simulink model "DinamicaCompleta"  (R2015a)
settings: Solver=ode45  StartTime=0.0  StopTime=10.0  RelTol=1e-3
values from neighbouring files (symbols this model uses):
  g = 1.6    [InitialParameters.m]
  M0 = 15000 - MFuel0    (= 7000)    [InitialParameters.m]
  MaxFl = 500    [InitialParameters.m]
  MaxFt = 44000    [InitialParameters.m]
  MFuel0 = 8000    [InitialParameters.m]
  Power = 3000    [InitialParameters.m]
  theta0 = 0    [InitialParameters.m]
  theta_dot0 = 0    [InitialParameters.m]
  x0 = 500    [InitialParameters.m]
  x_dot0 = 0    [InitialParameters.m]
  y0 = 160000    [InitialParameters.m]
  y_dot0 = -700    [InitialParameters.m]
settings Model: Creator=MateusVendramini  LastModifiedBy=MateusVendramini

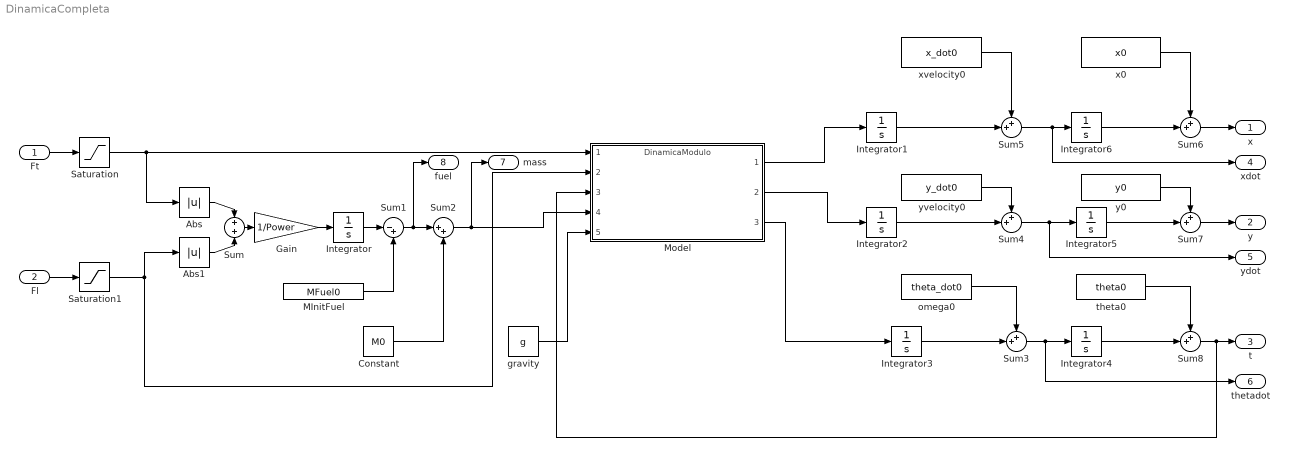
== system DinamicaCompleta ==
  Ft : Inport
  Fl : Inport  Port=2
  Abs : Abs
  Abs1 : Abs
  Constant : Constant  Value=M0
  Gain : Gain  Gain=1/Power
  Integrator{,1..6} (7 alike) : Integrator
  "MInitFuel " : Constant  Value=MFuel0
  Model : ModelReference  ModelNameDialog=DinamicaModulo.slx  SimulationMode=Normal  ModelReferenceVersion=1.3  CopyOfModelName=DinamicaModulo.slx  DefaultDataLogging=on
  Saturation : Saturate  UpperLimit=MaxFt  LowerLimit=-MaxFt
  Saturation1 : Saturate  UpperLimit=MaxFl  LowerLimit=-MaxFl
  Sum : Sum
  Sum1 : Sum  Inputs=|-+
  Sum2 : Sum  Inputs=|++
  Sum{3..8} (6 alike) : Sum  Inputs=++|
  gravity : Constant  Value=g
  omega0 : Constant  Value=theta_dot0
  theta0 : Constant  Value=theta0
  x0 : Constant  Value=x0
  xvelocity0 : Constant  Value=x_dot0
  y0 : Constant  Value=y0
  yvelocity0 : Constant  Value=y_dot0
  "x " : Outport
  "y " : Outport  Port=2
  "t " : Outport  Port=3
  "xdot " : Outport  Port=4
  "ydot " : Outport  Port=5
  "thetadot " : Outport  Port=6
  "mass " : Outport  Port=7
  "fuel " : Outport  Port=8
  wires:
  Ft/1 -> Saturation/1
  Fl/1 -> Saturation1/1
  Saturation/1 -> Model/1, Abs/1
  Abs/1 -> Sum/1
  Abs1/1 -> Sum/2
  Sum/1 -> Gain/1
  Gain/1 -> Integrator/1
  Integrator/1 -> Sum1/1
  "MInitFuel "/1 -> Sum1/2
  Sum1/1 -> "fuel "/1, Sum2/1
  Constant/1 -> Sum2/2
  Saturation1/1 -> Model/2, Abs1/1
  gravity/1 -> Model/5
  Model/1 -> Integrator1/1
  Model/2 -> Integrator2/1
  Model/3 -> Integrator3/1
  omega0/1 -> Sum3/1
  Integrator3/1 -> Sum3/2
  Sum3/1 -> "thetadot "/1, Integrator4/1
  Integrator2/1 -> Sum4/2
  yvelocity0/1 -> Sum4/1
  xvelocity0/1 -> Sum5/1
  Integrator1/1 -> Sum5/2
  Sum4/1 -> Integrator5/1, "ydot "/1
  Sum5/1 -> "xdot "/1, Integrator6/1
  x0/1 -> Sum6/1
  Integrator6/1 -> Sum6/2
  Integrator5/1 -> Sum7/2
  y0/1 -> Sum7/1
  theta0/1 -> Sum8/1
  Integrator4/1 -> Sum8/2
  Sum8/1 -> Model/3, "t "/1
  Sum7/1 -> "y "/1
  Sum6/1 -> "x "/1
  Sum2/1 -> "mass "/1, Model/4
